simulink model "AM"  (R2016a)
settings: Solver=VariableStepAuto  StartTime=0.0  StopTime=0.01  RelTol=1e-3
libraries: dsparch4 x1
settings Model: Creator=rashad  LastModifiedBy=rashad

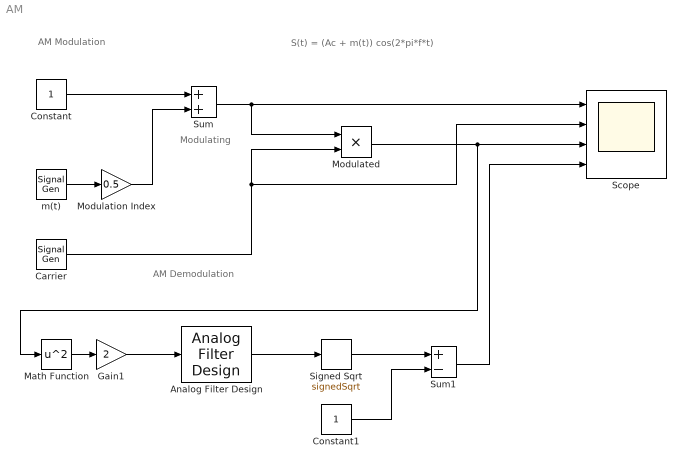
== system AM ==
  note: Modulating
  note: S(t) = (Ac + m(t)) cos(2*pi*f*t)
  note: AM Modulation
  note: AM Demodulation
  Analog Filter Design : dsparch4/Analog Filter Design  method=Butterworth  filttype=Lowpass  N=5  Wlo=2*pi*1000  Whi=80  Rp=2  Rs=40
  Carrier : SignalGenerator  Frequency=20000
  Constant : Constant
  Constant1 : Constant
  Gain1 : Gain  Gain=2
  Math Function : Math  Operator=square  SaturateOnIntegerOverflow=on
  Modulated : Product
  Modulation Index : Gain  Gain=0.5
  Scope : Scope  NumInputPorts=4
  Signed Sqrt : Sqrt  Operator=signedSqrt  SaturateOnIntegerOverflow=on
  Sum : Sum
  Sum1 : Sum  Inputs=+-
  m(t) : SignalGenerator  Frequency=1000
  wires:
  Constant/1 -> Sum/1
  Carrier/1 -> Scope/2, Modulated/2
  Modulation Index/1 -> Sum/2
  m(t)/1 -> Modulation Index/1
  Modulated/1 -> Math Function/1, Scope/3
  Sum/1 -> Scope/1, Modulated/1
  Math Function/1 -> Gain1/1
  Gain1/1 -> Analog Filter Design/1
  Analog Filter Design/1 -> Signed Sqrt/1
  Constant1/1 -> Sum1/2
  Signed Sqrt/1 -> Sum1/1
  Sum1/1 -> Scope/4
